simulink model "final_model_pid_thrust"  (R2015b)
settings: Solver=ode45  StartTime=0  StopTime=1000  FixedStep=0.001  RelTol=1e-3
libraries: simulink_extras x11, simulink x4, aerolibtransform2 x2, aerolibutil x2, aerolibobsolete x1, aerolibanim x1, aerolibasang x1
(part 2 of 2)

== system final_model_pid_thrust/Planta/Forces and Moments in Take-off/Taxiing2/Aerodynamic Forces /Lift/CL  ==
  CL0 : Inport
  CL_alpha : Inport  Port=2
  alpha : Inport  Port=3
  Add : Sum
  Product : Product
  "CL " : Outport
  wires:
  CL0/1 -> Add/1
  CL_alpha/1 -> Product/1
  Product/1 -> Add/2
  alpha/1 -> Product/2
  Add/1 -> "CL "/1

== system final_model_pid_thrust/Planta/Forces and Moments in Take-off/Taxiing2/Aerodynamic Forces /Lift/Lift ==
  V : Inport
  S : Inport  Port=2
  rho : Inport  Port=3
  CL : Inport  Port=4
  "0.5 " : Constant  Value=0.5
  Product : Product  Inputs=6
  L : Outport
  wires:
  rho/1 -> Product/2
  V/1 -> Product/4, Product/5
  CL/1 -> Product/6
  Product/1 -> L/1
  S/1 -> Product/3
  "0.5 "/1 -> Product/1

== system final_model_pid_thrust/Planta/Forces and Moments in Take-off/Taxiing2/Aerodynamic Moments / My/CM_A ==
  alpha : Inport
  delta : Inport  Port=2
  theta' : Inport  Port=3
  Add : Sum  Inputs=++++
  Cm0 : Constant  Value=0.04
  Cm_alpha : Constant  Value=-0.65
  Cm_delta : Constant  Value=-1.369
  Cm_q : Constant  Value=-15.20
  Product : Product
  Product1 : Product
  Product2 : Product
  CM_A : Outport
  wires:
  Product/1 -> Add/2
  Product1/1 -> Add/3
  Add/1 -> CM_A/1
  Cm_delta/1 -> Product1/1
  delta/1 -> Product1/2
  Cm0/1 -> Add/1
  Cm_alpha/1 -> Product/2
  alpha/1 -> Product/1
  Cm_q/1 -> Product2/1
  theta'/1 -> Product2/2
  Product2/1 -> Add/4

== system final_model_pid_thrust/Planta/Forces and Moments in Take-off/Taxiing2/Aerodynamic Moments / My/MA ==
  V : Inport
  S : Inport  Port=2
  rho_0 : Inport  Port=3
  CM_A : Inport  Port=4
  c : Inport  Port=5
  "0.5 " : Constant  Value=0.5
  Product : Product  Inputs=7
  MA : Outport
  wires:
  rho_0/1 -> Product/2
  V/1 -> Product/5, Product/4
  CM_A/1 -> Product/7
  Product/1 -> MA/1
  S/1 -> Product/3
  "0.5 "/1 -> Product/1
  c/1 -> Product/6

== system final_model_pid_thrust/Planta/Forces and Moments in Take-off/Transition/Aerodynamic Forces /Drag/CD ==
  CD0 : Inport
  k : Inport  Port=2
  CL : Inport  Port=3
  Add : Sum
  Product : Product  Inputs=3
  CD : Outport
  wires:
  CD0/1 -> Add/1
  Product/1 -> Add/2
  k/1 -> Product/1
  Add/1 -> CD/1
  CL/1 -> Product/3, Product/2

== system final_model_pid_thrust/Planta/Forces and Moments in Take-off/Transition/Aerodynamic Forces /Drag/Drag ==
  V : Inport
  S : Inport  Port=2
  rho : Inport  Port=3
  CD : Inport  Port=4
  "0.5 " : Constant  Value=0.5
  Product : Product  Inputs=6
  D : Outport
  wires:
  rho/1 -> Product/2
  V/1 -> Product/4, Product/5
  CD/1 -> Product/6
  Product/1 -> D/1
  S/1 -> Product/3
  "0.5 "/1 -> Product/1

== system final_model_pid_thrust/Planta/Forces and Moments in Take-off/Transition/Aerodynamic Forces /Fy equation/Dynamic pressure  ==
  V : Inport
  "rho " : Inport  Port=2
  Constant : Constant  Value=0.5
  Math Function : Math  Operator=square  SaturateOnIntegerOverflow=on
  Product : Product  Inputs=3
  q : Outport
  wires:
  Math Function/1 -> Product/1
  "rho "/1 -> Product/3
  Product/1 -> q/1
  Constant/1 -> Product/2
  V/1 -> Math Function/1

== system final_model_pid_thrust/Planta/Forces and Moments in Take-off/Transition/Aerodynamic Forces /Fy equation/Lateral Force Coefficient ==
  "beta " : Inport
  delta_a : Inport  Port=2
  delta_r : Inport  Port=3
  C_Y0 : Constant  Value=0
  C_Ybeta : Constant  Value=-0.404
  C_Ydelta_a : Constant  Value=0
  C_Ydelta_r : Constant  Value=0.187
  Product1 : Product
  Product2 : Product
  Product3 : Product
  "Sum " : Sum  Inputs=++++
  C_Y : Outport
  wires:
  "beta "/1 -> Product1/1
  C_Ybeta/1 -> Product1/2
  delta_a/1 -> Product2/1
  C_Ydelta_a/1 -> Product2/2
  delta_r/1 -> Product3/1
  C_Ydelta_r/1 -> Product3/2
  C_Y0/1 -> "Sum "/1
  Product1/1 -> "Sum "/2
  Product2/1 -> "Sum "/3
  Product3/1 -> "Sum "/4
  "Sum "/1 -> C_Y/1

== system final_model_pid_thrust/Planta/Forces and Moments in Take-off/Transition/Aerodynamic Forces /Lift/CL  ==
  CL0 : Inport
  CL_alpha : Inport  Port=2
  alpha : Inport  Port=3
  Add : Sum
  Product : Product
  "CL " : Outport
  wires:
  CL0/1 -> Add/1
  CL_alpha/1 -> Product/1
  Product/1 -> Add/2
  alpha/1 -> Product/2
  Add/1 -> "CL "/1

== system final_model_pid_thrust/Planta/Forces and Moments in Take-off/Transition/Aerodynamic Forces /Lift/Lift ==
  V : Inport
  S : Inport  Port=2
  rho : Inport  Port=3
  CL : Inport  Port=4
  "0.5 " : Constant  Value=0.5
  Product : Product  Inputs=6
  L : Outport
  wires:
  rho/1 -> Product/2
  V/1 -> Product/4, Product/5
  CL/1 -> Product/6
  Product/1 -> L/1
  S/1 -> Product/3
  "0.5 "/1 -> Product/1

== system final_model_pid_thrust/Planta/Forces and Moments in Take-off/Transition/Aerodynamic Moments /Pitch Moment/C_mA ==
  alpha : Inport
  delta_e : Inport  Port=2
  theta' : Inport  Port=3
  Add : Sum  Inputs=++++
  C_m0 : Constant  Value=0.04
  C_malpha : Constant  Value=-0.65
  C_mdelta_e : Constant  Value=-1.369
  C_mq : Constant  Value=-15.20
  Product : Product
  Product1 : Product
  Product2 : Product
  C_mA : Outport
  wires:
  Product/1 -> Add/2
  Product1/1 -> Add/3
  Add/1 -> C_mA/1
  C_mdelta_e/1 -> Product1/1
  delta_e/1 -> Product1/2
  C_m0/1 -> Add/1
  C_malpha/1 -> Product/2
  alpha/1 -> Product/1
  C_mq/1 -> Product2/1
  theta'/1 -> Product2/2
  Product2/1 -> Add/4

== system final_model_pid_thrust/Planta/Forces and Moments in Take-off/Transition/Aerodynamic Moments /Pitch Moment/Pitch Moment ==
  C_mA : Inport
  V : Inport  Port=2
  rho : Inport  Port=3
  S : Inport  Port=4
  c : Inport  Port=5
  "0.5 " : Constant  Value=0.5
  Product : Product  Inputs=7
  M_A : Outport
  wires:
  rho/1 -> Product/2
  V/1 -> Product/4, Product/5
  C_mA/1 -> Product/7
  Product/1 -> M_A/1
  S/1 -> Product/3
  "0.5 "/1 -> Product/1
  c/1 -> Product/6

== system final_model_pid_thrust/Planta/Forces and Moments in Take-off/Transition/Aerodynamic Moments /Roll Moment/Dynamic pressure  ==
  V : Inport
  "rho " : Inport  Port=2
  Constant : Constant  Value=0.5
  Math Function : Math  Operator=square  SaturateOnIntegerOverflow=on
  Product : Product  Inputs=3
  q : Outport
  wires:
  Math Function/1 -> Product/1
  "rho "/1 -> Product/3
  Product/1 -> q/1
  Constant/1 -> Product/2
  V/1 -> Math Function/1

== system final_model_pid_thrust/Planta/Forces and Moments in Take-off/Transition/Aerodynamic Moments /Roll Moment/Roll Moment Coefficient ==
  "beta " : Inport
  delta_a : Inport  Port=2
  delta_r : Inport  Port=3
  C_l0 : Constant  Value=0
  C_lbeta : Constant  Value=-0.0895
  C_ldelta_a : Constant  Value=0.2290
  C_ldelta_r : Constant  Value=0.0147
  Product1 : Product
  Product2 : Product
  Product3 : Product
  "Sum " : Sum  Inputs=++++
  C_l : Outport
  wires:
  "beta "/1 -> Product1/1
  C_lbeta/1 -> Product1/2
  delta_a/1 -> Product2/1
  C_ldelta_a/1 -> Product2/2
  delta_r/1 -> Product3/1
  C_ldelta_r/1 -> Product3/2
  C_l0/1 -> "Sum "/1
  Product1/1 -> "Sum "/2
  Product2/1 -> "Sum "/3
  Product3/1 -> "Sum "/4
  "Sum "/1 -> C_l/1

== system final_model_pid_thrust/Planta/Forces and Moments in Take-off/Transition/Aerodynamic Moments /Yaw Moment/Dynamic pressure  ==
  V : Inport
  "rho " : Inport  Port=2
  Constant : Constant  Value=0.5
  Math Function : Math  Operator=square  SaturateOnIntegerOverflow=on
  Product : Product  Inputs=3
  q : Outport
  wires:
  Math Function/1 -> Product/1
  "rho "/1 -> Product/3
  Product/1 -> q/1
  Constant/1 -> Product/2
  V/1 -> Math Function/1

== system final_model_pid_thrust/Planta/Forces and Moments in Take-off/Transition/Aerodynamic Moments /Yaw Moment/Yaw Moment Coefficient ==
  "beta " : Inport
  delta_a : Inport  Port=2
  delta_r : Inport  Port=3
  C_n0 : Constant  Value=0
  C_nbeta : Constant  Value=0.0907
  C_ndelta_a : Constant  Value=-0.0504
  C_ndelta_r : Constant  Value=-0.0805
  Product1 : Product
  Product2 : Product
  Product3 : Product
  "Sum " : Sum  Inputs=++++
  C_n : Outport
  wires:
  "beta "/1 -> Product1/1
  C_nbeta/1 -> Product1/2
  delta_a/1 -> Product2/1
  C_ndelta_a/1 -> Product2/2
  delta_r/1 -> Product3/1
  C_ndelta_r/1 -> Product3/2
  C_n0/1 -> "Sum "/1
  Product1/1 -> "Sum "/2
  Product2/1 -> "Sum "/3
  Product3/1 -> "Sum "/4
  "Sum "/1 -> C_n/1
